simulink model "pdl_linear_hw4hybrid"  (R2017a)
settings: Solver=FixedStepAuto  StartTime=0.0  StopTime=duration  FixedStep=Ts  RelTol=1e-3
values from neighbouring files (symbols this model uses):
  A_a = [A E*Cw; zeros(2,4) Aw]    [pendulum_hw4linear.m]
  B_a = [B; zeros(2,1)]    [pendulum_hw4linear.m]
  C_a = [C zeros(2,2)]    [pendulum_hw4linear.m]
  E_a = [zeros(4,2); Bw]    [pendulum_hw4linear.m]
  f_p = 1e-4    (= 0.0001)    [pendulum_hw4linear.m]    (also in pendulum_hw4nonlinear.m)
  LC1_D = c2d(LC1_C,Ts)    [localcontroller.m]
  LC2_D = c2d(LC2_C,Ts)    [localcontroller.m]
  LC3_D = c2d(LC3_C,Ts)    [localcontroller.m]
  LC4_D = c2d(LC4_C,Ts)    [localcontroller.m]
  m_p = 1e-7    (= 1e-07)    [pendulum_hw4linear.m]    (also in pendulum_hw4nonlinear.m)
  Q_k = 1e3*diag([10,1e-4])    [pendulum_hw4linear.m]    (also in pendulum_hw4nonlinear.m = diag([1 1]))
  R_k = 1.0015e-4*diag([1 1])    [pendulum_hw4linear.m]    (also in pendulum_hw4nonlinear.m = 1e-4*diag([1 1]))
  Ts = 0.001    [localcontroller.m]    (also in pendulum_hw4linear.m; pendulum_hw4nonlinear.m)
  w_p = 10    [pendulum_hw4linear.m]    (also in pendulum_hw4nonlinear.m)
  X_0 = [0;0*pi/180;0;0;0;0]    [pendulum_hw4linear.m]    (also in pendulum_hw4nonlinear.m = [0;0*pi/180;0;0])
undefined symbols (not defined in the file or in its folder): Delta_1, Delta_2, Delta_3, Delta_4, Gamma_1, Gamma_2, Gamma_3, Gamma_4, Phi_1, Phi_2, Phi_3, Phi_4
libraries: simulink x3
settings Model: Creator=Salmon  LastModifiedBy=Salmon

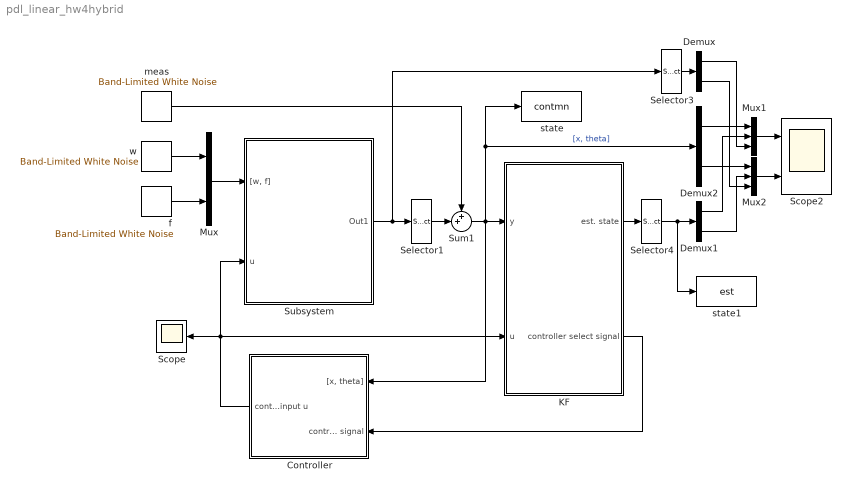
== system pdl_linear_hw4hybrid ==
  Controller : Subsystem
  Demux : Demux  Outputs=2
  Demux1 : Demux  Outputs=2
  Demux2 : Demux  Outputs=2
  KF : Subsystem
  Mux : Mux  Inputs=2
  Mux1 : Mux  Inputs=3
  Mux2 : Mux  Inputs=3
  Scope : Scope
  Scope2 : Scope  NumInputPorts=2
  Selector1 : Selector  InputPortWidth=6  IndexOptions=Index vector (dialog)  Indices=[1 2]  OutputSizes=1
  Selector3 : Selector  InputPortWidth=6  IndexOptions=Index vector (dialog)  Indices=[1 2]  OutputSizes=1
  Selector4 : Selector  InputPortWidth=6  IndexOptions=Index vector (dialog)  Indices=[1 2]  OutputSizes=1
  Subsystem : Subsystem
  Sum1 : Sum  Inputs=++|
  f : simulink/Sources/Band-Limited White Noise  Cov=[f_p]  Ts=Ts  seed=[23341]
  meas : simulink/Sources/Band-Limited White Noise  Cov=[m_p,m_p]  Ts=Ts  seed=[123,23341]
  state : ToWorkspace  VariableName=contmn  SaveFormat=Structure With Time  SampleTime=Ts
  state1 : ToWorkspace  VariableName=est  SaveFormat=Structure With Time  SampleTime=Ts
  w : simulink/Sources/Band-Limited White Noise  Cov=[w_p]  Ts=Ts  seed=[23341]
  wires:
  w/1 -> Mux/1
  f/1 -> Mux/2
  Mux/1 -> Subsystem/1("[w, f]")
  Subsystem/1(Out1) -> Selector1/1, Selector3/1
  Demux/1 -> Mux1/3
  Demux/2 -> Mux2/3
  Selector1/1 -> Sum1/2
  Demux1/1 -> Mux1/2
  KF/2(controller select signal) -> Controller/2(controller select signal)
  Demux1/2 -> Mux2/2
  meas/1 -> Sum1/1
  Demux2/1 -> Mux1/1
  Demux2/2 -> Mux2/1
  Mux1/1 -> Scope2/1
  Mux2/1 -> Scope2/2
  Sum1/1 -> Controller/1("[x, theta]"), KF/1(y), state/1, Demux2/1  "[x, theta]"
  Selector3/1 -> Demux/1
  Selector4/1 -> state1/1, Demux1/1
  Controller/1(control input u) -> Subsystem/2(u), KF/2(u), Scope/1
  KF/1(est. state) -> Selector4/1

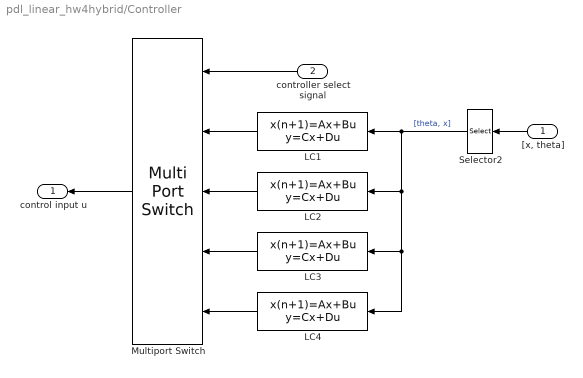
== system pdl_linear_hw4hybrid/Controller ==
  "[x, theta]" : Inport
  controller select signal : Inport  Port=2
  LC1 : DiscreteStateSpace  A=LC1_D.A  B=LC1_D.B  C=LC1_D.C  D=LC1_D.D  SampleTime=Ts
  LC2 : DiscreteStateSpace  A=LC2_D.A  B=LC2_D.B  C=LC2_D.C  D=LC2_D.D  SampleTime=Ts
  LC3 : DiscreteStateSpace  A=LC3_D.A  B=LC3_D.B  C=LC3_D.C  D=LC3_D.D  SampleTime=Ts
  LC4 : DiscreteStateSpace  A=LC4_D.A  B=LC4_D.B  C=LC4_D.C  D=LC4_D.D  SampleTime=Ts
  Multiport Switch : MultiPortSwitch  Inputs=4  DiagnosticForDefault=None
  Selector2 : Selector  InputPortWidth=2  IndexOptions=Index vector (dialog)  Indices=[2 1]  OutputSizes=1
  control input u : Outport
  wires:
  LC4/1 -> Multiport Switch/5
  controller select signal/1 -> Multiport Switch/1
  LC3/1 -> Multiport Switch/4
  LC2/1 -> Multiport Switch/3
  LC1/1 -> Multiport Switch/2
  Selector2/1 -> LC4/1, LC3/1, LC2/1, LC1/1  "[theta, x]"
  Multiport Switch/1 -> control input u/1
  "[x, theta]"/1 -> Selector2/1

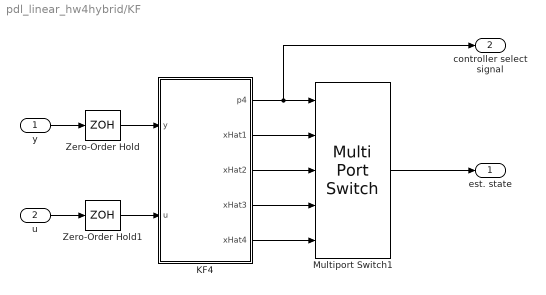
== system pdl_linear_hw4hybrid/KF ==
  y : Inport
  u : Inport  Port=2
  KF4 : Subsystem
  Multiport Switch1 : MultiPortSwitch  Inputs=4  DiagnosticForDefault=None
  Zero-Order Hold : ZeroOrderHold  SampleTime=Ts
  Zero-Order Hold1 : ZeroOrderHold  SampleTime=Ts
  est. state : Outport
  controller select signal : Outport  Port=2
  wires:
  u/1 -> Zero-Order Hold1/1
  Multiport Switch1/1 -> est. state/1
  y/1 -> Zero-Order Hold/1
  KF4/5("xHat4 ") -> Multiport Switch1/5
  KF4/4(xHat3) -> Multiport Switch1/4
  KF4/3(xHat2) -> Multiport Switch1/3
  KF4/2(xHat1) -> Multiport Switch1/2
  KF4/1(p4) -> controller select signal/1, Multiport Switch1/1
  Zero-Order Hold/1 -> KF4/1(y)
  Zero-Order Hold1/1 -> KF4/2(u)

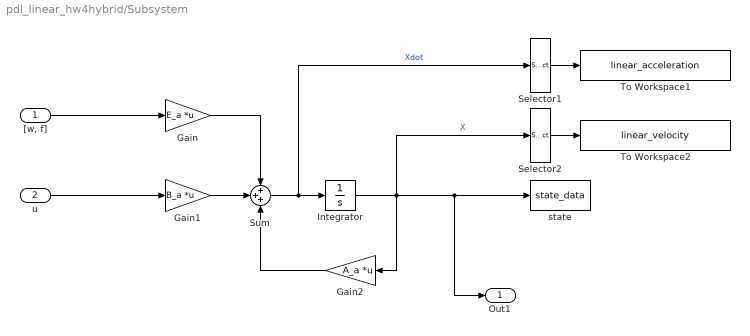
== system pdl_linear_hw4hybrid/Subsystem ==
  "[w, f]" : Inport
  u : Inport  Port=2
  Gain : Gain  Gain=E_a  Multiplication=Matrix(K*u)
  Gain1 : Gain  Gain=B_a  Multiplication=Matrix(K*u)
  Gain2 : Gain  Gain=A_a  Multiplication=Matrix(K*u)
  Integrator : Integrator  InitialCondition=X_0
  Selector1 : Selector  InputPortWidth=6  IndexOptions=Index vector (dialog)  Indices=[3]  OutputSizes=1
  Selector2 : Selector  InputPortWidth=6  IndexOptions=Index vector (dialog)  Indices=[3]  OutputSizes=1
  Sum : Sum  Inputs=+++
  To Workspace1 : ToWorkspace  VariableName=linear_acceleration  SaveFormat=Structure With Time  SampleTime=-1
  To Workspace2 : ToWorkspace  VariableName=linear_velocity  SaveFormat=Structure With Time  SampleTime=-1
  state : ToWorkspace  VariableName=state_data  SaveFormat=Structure With Time  SampleTime=Ts
  Out1 : Outport
  wires:
  "[w, f]"/1 -> Gain/1
  Gain/1 -> Sum/1
  Gain1/1 -> Sum/2
  Selector2/1 -> To Workspace2/1
  Selector1/1 -> To Workspace1/1
  Gain2/1 -> Sum/3
  u/1 -> Gain1/1
  Integrator/1 -> Gain2/1, Selector2/1, Out1/1, state/1  "X"
  Sum/1 -> Integrator/1, Selector1/1  "Xdot"

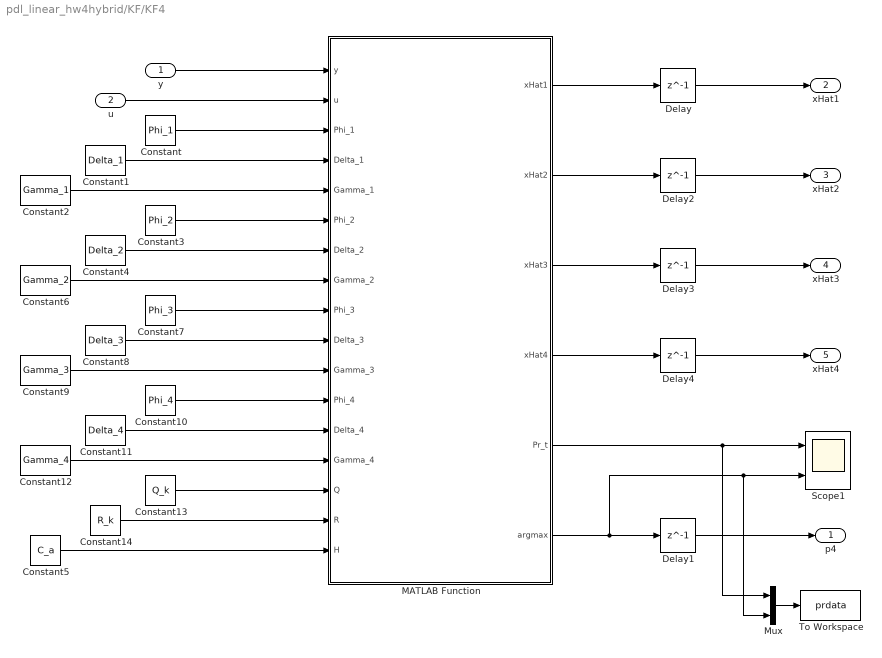
== system pdl_linear_hw4hybrid/KF/KF4 ==
  y : Inport
  u : Inport  Port=2
  Constant : Constant  Value=Phi_1
  Constant1 : Constant  Value=Delta_1
  Constant10 : Constant  Value=Phi_4
  Constant11 : Constant  Value=Delta_4
  Constant12 : Constant  Value=Gamma_4
  Constant13 : Constant  Value=Q_k
  Constant14 : Constant  Value=R_k
  Constant2 : Constant  Value=Gamma_1
  Constant3 : Constant  Value=Phi_2
  Constant4 : Constant  Value=Delta_2
  Constant5 : Constant  Value=C_a
  Constant6 : Constant  Value=Gamma_2
  Constant7 : Constant  Value=Phi_3
  Constant8 : Constant  Value=Delta_3
  Constant9 : Constant  Value=Gamma_3
  Delay{,1..4} (5 alike) : Delay  DelayLength=1  InitialCondition=0
  MATLAB Function : MATLAB Function  TreatAsAtomicUnit=on
  Mux : Mux  Inputs=2
  Scope1 : Scope  NumInputPorts=2
  To Workspace : ToWorkspace  VariableName=prdata  SaveFormat=Structure With Time  SampleTime=-1
  p4 : Outport
  xHat1 : Outport  Port=2
  xHat2 : Outport  Port=3
  xHat3 : Outport  Port=4
  "xHat4 " : Outport  Port=5
  wires:
  MATLAB Function/1(xHat1) -> Delay/1
  Constant5/1 -> MATLAB Function/17(H)
  Delay/1 -> xHat1/1
  Constant1/1 -> MATLAB Function/4(Delta_1)
  Constant/1 -> MATLAB Function/3(Phi_1)
  Constant2/1 -> MATLAB Function/5(Gamma_1)
  u/1 -> MATLAB Function/2(u)
  y/1 -> MATLAB Function/1(y)
  Delay1/1 -> p4/1
  MATLAB Function/6(argmax) -> Mux/2, Scope1/2, Delay1/1
  MATLAB Function/2(xHat2) -> Delay2/1
  Delay2/1 -> xHat2/1
  MATLAB Function/3(xHat3) -> Delay3/1
  Delay3/1 -> xHat3/1
  MATLAB Function/4(xHat4) -> Delay4/1
  Delay4/1 -> "xHat4 "/1
  MATLAB Function/5(Pr_t) -> Mux/1, Scope1/1
  Constant3/1 -> MATLAB Function/6(Phi_2)
  Constant6/1 -> MATLAB Function/8(Gamma_2)
  Constant4/1 -> MATLAB Function/7(Delta_2)
  Constant7/1 -> MATLAB Function/9(Phi_3)
  Constant9/1 -> MATLAB Function/11(Gamma_3)
  Constant8/1 -> MATLAB Function/10(Delta_3)
  Constant10/1 -> MATLAB Function/12(Phi_4)
  Constant12/1 -> MATLAB Function/14(Gamma_4)
  Constant11/1 -> MATLAB Function/13(Delta_4)
  Constant13/1 -> MATLAB Function/15(Q)
  Constant14/1 -> MATLAB Function/16(R)
  Mux/1 -> To Workspace/1

== matlab function pdl_linear_hw4hybrid/KF/KF4/MATLAB Function ==
  data: y input; u input; xHat1 output; xHat2 output; xHat3 output; xHat4 output; Pr_t output; Phi_1 input; Delta_1 input; Gamma_1 input; Phi_2 input; Delta_2 input; Gamma_2 input; Phi_3 input; Delta_3 input; Gamma_3 input; Phi_4 input; Delta_4 input; Gamma_4 input; Q input; R input; H input; argmax output
function [xHat1,xHat2,xHat3,xHat4,Pr_t,argmax] = fcn(y,u,Phi_1,Delta_1,Gamma_1,Phi_2,Delta_2,Gamma_2,Phi_3,Delta_3,Gamma_3,Phi_4,Delta_4,Gamma_4,Q,R,H)

%persistent Pbar 
persistent xbar1 Sig1 Pr1 
persistent xbar2 Sig2 Pr2
persistent xbar3 Sig3 Pr3
persistent xbar4 Sig4 Pr4

if isempty(xbar1) xbar1 = zeros(6,1);  end

if isempty(Sig1)  Sig1 = 1e-18*eye(6);  end

if isempty(Pr1)   Pr1 = 0.25;   end

if isempty(xbar2) xbar2 = zeros(6,1);  end

if isempty(Sig2)  Sig2 = 1e-18*eye(6);  end

if isempty(Pr2)   Pr2 = 0.25;   end

if isempty(xbar3) xbar3 = zeros(6,1);  end

if isempty(Sig3)  Sig3 = 1e-18*eye(6);  end

if isempty(Pr3)   Pr3 = 0.25;   end

if isempty(xbar4) xbar4 = zeros(6,1);  end

if isempty(Sig4)  Sig4 = 1e-18*eye(6);  end

if isempty(Pr4)   Pr4 = 0.25;   end

% KF1
K_hi1 = Sig1*H'*(H*Sig1*H'+R)^(-1);
y_o1 = H*xbar1;
y_e1 = y-y_o1;
Sig_hat1 = (eye(6)-K_hi1*H)*Sig1*(eye(6)-K_hi1*H)'+K_hi1*R*K_hi1';
xHat1 = xbar1 + K_hi1*y_e1;
xbar1 = Phi_1*xHat1+Delta_1*u;
Sig1 = Phi_1*Sig_hat1*Phi_1'+Gamma_1*Q*Gamma_1';
S_hi1 = H*Sig1*H' + R;

Pr_numerator1 = exp(-0.5*y_e1'*S_hi1^(-1)*y_e1)*Pr1*(sqrt((2*pi)^2*det(S_hi1)))^(-1);

% KF2
K_hi2 = Sig2*H'*(H*Sig2*H'+R)^(-1);
y_o2 = H*xbar2;
y_e2 = y-y_o2;
Sig_hat2 = (eye(6)-K_hi2*H)*Sig2*(eye(6)-K_hi2*H)'+K_hi2*R*K_hi2';
xHat2 = xbar2 + K_hi2*y_e2;
xbar2 = Phi_2*xHat2+Delta_2*u;
Sig2 = Phi_2*Sig_hat2*Phi_2'+Gamma_2*Q*Gamma_2';
S_hi2 = H*Sig2*H' + R;

Pr_numerator2 = exp(-0.5*y_e2'*S_hi2^(-1)*y_e2)*Pr2*(sqrt((2*pi)^2*det(S_hi2)))^(-1);

% KF3
K_hi3 = Sig3*H'*(H*Sig3*H'+R)^(-1);
y_o3 = H*xbar3;
y_e3 = y-y_o3;
Sig_hat3 = (eye(6)-K_hi3*H)*Sig3*(eye(6)-K_hi3*H)'+K_hi3*R*K_hi3';
xHat3 = xbar3 + K_hi3*y_e3;
xbar3 = Phi_3*xHat3+Delta_3*u;
Sig3 = Phi_3*Sig_hat3*Phi_3'+Gamma_3*Q*Gamma_3';
S_hi3 = H*Sig3*H' + R;

Pr_numerator3 = exp(-0.5*y_e3'*S_hi3^(-1)*y_e3)*Pr3*(sqrt((2*pi)^2*det(S_hi3)))^(-1);

% KF4
K_hi4 = Sig4*H'*(H*Sig4*H'+R)^(-1);
y_o4 = H*xbar4;
y_e4 = y-y_o4;
Sig_hat4 = (eye(6)-K_hi4*H)*Sig4*(eye(6)-K_hi4*H)'+K_hi4*R*K_hi4';
xHat4 = xbar4 + K_hi4*y_e4;
xbar4 = Phi_4*xHat4+Delta_4*u;
Sig4 = Phi_4*Sig_hat4*Phi_4'+Gamma_4*Q*Gamma_4';
S_hi4 = H*Sig4*H' + R;

Pr_numerator4 = exp(-0.5*y_e4'*S_hi4^(-1)*y_e4)*Pr4*(sqrt((2*pi)^2*det(S_hi4)))^(-1);

% Calculate conditional probabilities
Pr_denom = Pr_numerator1 + Pr_numerator2 + Pr_numerator3 + Pr_numerator4;
Pr1 = Pr_numerator1/Pr_denom;
Pr2 = Pr_numerator2/Pr_denom;
Pr3 = Pr_numerator3/Pr_denom;
Pr4 = Pr_numerator4/Pr_denom;

Pr_t = [Pr1,Pr2,Pr3,Pr4];

% Maximum likelihood
[~,argmax] = max(Pr_t);
